simulink model "CytronSubsystem"  (R2017a)
settings: Solver=VariableStepAuto  StartTime=0.0  StopTime=10.0  RelTol=1e-3
libraries: arduinolib x4
settings Model: Creator=Rutvik  LastModifiedBy=Rutvik

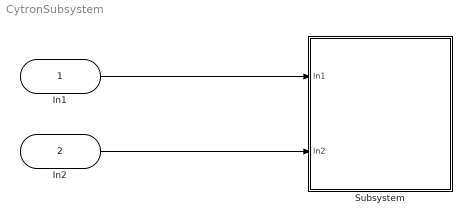
== system CytronSubsystem ==
  In1 : Inport
  In2 : Inport  Port=2
  Subsystem : Subsystem
  wires:
  In1/1 -> Subsystem/1(In1)
  In2/1 -> Subsystem/2(In2)

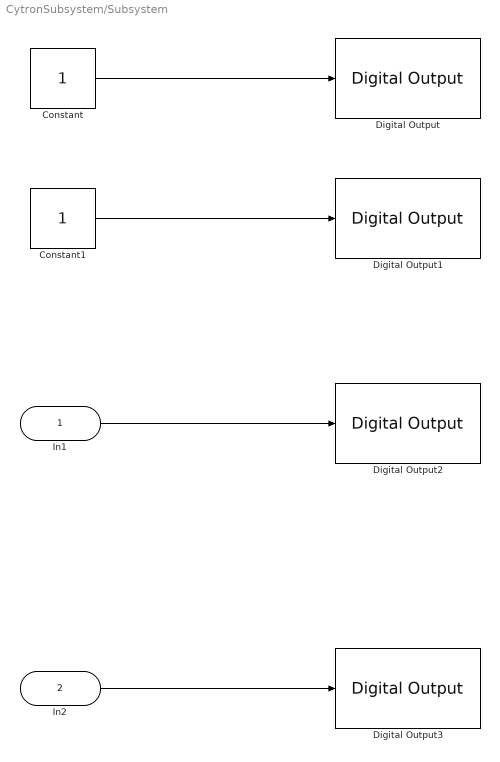
== system CytronSubsystem/Subsystem ==
  In1 : Inport
  In2 : Inport  Port=2
  Constant : Constant
  Constant1 : Constant
  Digital Output : arduinolib/Digital Output  pinNumber=10
  Digital Output1 : arduinolib/Digital Output  pinNumber=11
  Digital Output2 : arduinolib/Digital Output  pinNumber=12
  Digital Output3 : arduinolib/Digital Output  pinNumber=13
  wires:
  In1/1 -> Digital Output2/1
  Constant1/1 -> Digital Output1/1
  Constant/1 -> Digital Output/1
  In2/1 -> Digital Output3/1
